simulink library "aeroblk_lib_HL20"  (Simulink 6.0)
settings: Solver=ode45  SolverMode=SingleTasking  StartTime=0.0  StopTime=10.0  RelTol=1e-3
values from neighbouring files (symbols this model uses):
  a_matrix = [-0.028840208852 -0.0156596305643 -0.0560912779756 -0.0863202941854 0.0209519994416 0.0112571762889 23.9049039727 0 2.90446405277 0 -10.5841662935 0 ... (11560 elements, 17x17x8x5)]    [aeroblk_HL20_autopilot_gains.mat]
  A_matrix = [-0.028840208852 -0.0156596305643 -0.0560912779756 -0.0863202941854 0.0209519994416 0.0112571762889 0 0 0 0 0 0 ... (11560 elements, 17x17x8x5)]    [aeroblk_HL20_autopilot_gains.mat]
  alpha_vec_Cn0 = [-10 -5 0 5 10 15 20 25 30]    [aeroblk_init_HL20.m]
  b_matrix = [-0.0157218860845 -0.283968320777 0.321370128412 0.271058535159 0.0185568065093 -0.00784369239396 -0.320886300542 1.82463546416 -0.0471251877299 0.142152392032 -0.0609086167769 0.505612659091 ... (2040 elements, 17x3x8x5)]    [aeroblk_HL20_autopilot_gains.mat]
  B_matrix = [0 0 0 0 0 0 4 0 0 0 0 0 ... (2040 elements, 17x3x8x5)]    [aeroblk_HL20_autopilot_gains.mat]
  b_ref = 13.89/m2ft    (= 4.23367186452)    [aeroblk_init_HL20.m]
  beta_vec_Cn0 = [0 2 5 10]    [aeroblk_init_HL20.m]
  c_matrix = [-5.97622599319 -0.726116013193 2.64604157338 -40.7494939461 11.661494324 21.0342779763 20.6745716213 -19.9416021106 -13.12545371 926.002157715 -187.969629212 -231.434488107 ... (2040 elements, 3x17x8x5)]    [aeroblk_HL20_autopilot_gains.mat]
  C_matrix = [0 0 0 0 0 0 0 0 0 -58.994812472 0 0 ... (2040 elements, 3x17x8x5)]    [aeroblk_HL20_autopilot_gains.mat]
  Clbeta = -0.00787    [aeroblk_init_HL20.m]
  Cm0 = reshape(temp(:,2),length(beta_vec_0),length(alpha_vec_0))    [aeroblk_init_HL20.m]
  CX0 = -reshape(temp(:,3),length(beta_vec_0),length(alpha_vec_0))    [aeroblk_init_HL20.m]
  CYbeta = -0.01242    [aeroblk_init_HL20.m]
  CZ0 = -reshape(temp(:,1),length(beta_vec_0),length(alpha_vec_0))    [aeroblk_init_HL20.m]
  d_matrix = [0 0 0 0 0 0 0 0 0 0 0 0 ... (360 elements, 3x3x8x5)]    [aeroblk_HL20_autopilot_gains.mat]
  d_ref = 0.75/m2ft    (= 0.228599992685)    [aeroblk_guid_dat.m]    (also in aeroblk_init_HL20.m = 8.60755172456)
  F_matrix = [5.97622599319 0.726116013193 -2.64604157338 40.7494939461 -11.661494324 -21.0342779763 -20.6745716213 19.9416021106 13.12545371 -926.002157715 187.969629212 231.434488107 ... (2040 elements, 3x17x8x5)]    [aeroblk_HL20_autopilot_gains.mat]
  H_matrix = [-0.0157218860845 -0.283968320777 0.321370128412 0.271058535159 0.0185568065093 -0.00784369239396 -0.320886300542 1.82463546416 -0.0471251877299 0.142152392032 -0.0609086167769 0.505612659091 ... (2040 elements, 17x3x8x5)]    [aeroblk_HL20_autopilot_gains.mat]
  mass = 13.98/Kg2slug    (= 204.022661401)    [aeroblk_guid_dat.m]    (also in aeroblk_init_HL20.m = 11738.9844962)
  x_cg = 0.575*len_veh    (= 4.78635044684)    [aeroblk_init_HL20.m]
  x_ref = 0.54*len_veh    (= 4.49500737616)    [aeroblk_init_HL20.m]
undefined symbols (not defined in the file or in its folder): F, Light, MIL
libraries: simulink x60, aerolibconvert x4, aerolibschedule x4, aerolibasang x3, aerolibwind2 x3, aeroblk_lib_HL20 x1, aerolib6dof2 x1, aerolibatmos2 x1, aerolibgravity2 x1, aerolibadyn x1
(part 2 of 2)

== system aeroblk_lib_HL20/HL20 Airframe/Aerodynamic Coefficients/Body Rate Damping/q ==
  Alpha : Inport  Port=1  LatchInput=off
  Cmq : simulink/Lookup Tables/Interpolation (n-D) using PreLookup  numDimsPopupSelect=1  explicitNumDims=2  table=Cmq  interpMethod=Linear  extrapMethod=Linear  rangeErrorMode=None  NumSelectionDims=0
  Constant3 : Constant  Value=0
  Mux1 : Mux  Inputs=6
  delCoeff : Outport
  wires:
  Cmq/1 -> Mux1/5
  Constant3/1 -> Mux1/1, Mux1/2, Mux1/3, Mux1/6, Mux1/4
  Mux1/1 -> delCoeff/1
  Alpha/1 -> Cmq/1

== system aeroblk_lib_HL20/HL20 Airframe/Aerodynamic Coefficients/Body Rate Damping/r ==
  Alpha : Inport  Port=1  LatchInput=off
  Clr : simulink/Lookup Tables/Interpolation (n-D) using PreLookup  numDimsPopupSelect=1  explicitNumDims=2  table=Clr  interpMethod=Linear  extrapMethod=Linear  rangeErrorMode=None  NumSelectionDims=0
  Cnr : simulink/Lookup Tables/Interpolation (n-D) using PreLookup  numDimsPopupSelect=1  explicitNumDims=2  table=Cnr  interpMethod=Linear  extrapMethod=Linear  rangeErrorMode=None  NumSelectionDims=0
  Constant : Constant  Value=0
  Mux1 : Mux  Inputs=6
  delCoeff : Outport
  wires:
  Cnr/1 -> Mux1/6
  Clr/1 -> Mux1/4  "Cl"
  Constant/1 -> Mux1/1, Mux1/2, Mux1/5, Mux1/3  "Cxr"
  Mux1/1 -> delCoeff/1
  Alpha/1 -> Clr/1, Cnr/1
